simulink model "angle_led"  (R2021b)
settings: Solver=FixedStepDiscrete  StartTime=0.0  StopTime=inf  FixedStep=0.0005  RelTol=1e-3
libraries: simulink x4
settings Model: Creator=ysl  LastModifiedBy=ysl
settings OptimizationCC: DefaultParameterBehavior=Inlined  EnhancedBackFolding=on  PassReuseOutputArgsAs=Individual arguments  ZeroExternalMemoryAtStartup=off  ZeroInternalMemoryAtStartup=off  OptimizeBlockOrder=speed  DifferentSizesBufferReuse=on  OptimizationCustomize=off  EfficientTunableParamExpr=on
settings DebuggingCC: ParameterTunabilityLossMsg=error
settings SFSimCC: MATLABDynamicMemAlloc=off
settings RTWCC: Description=IFR StackLite-DualDrive Base on stm32f405RGT6  SystemTargetFile=stacklite_dualdrive.tlc  TemplateMakefile=stacklite_dualdrive.tmf  GenerateReport=on
settings CodeAppCC: ForceParamTrailComments=on  IgnoreCustomStorageClasses=off  OperatorAnnotations=on  SimulinkDataObjDesc=on  SFDataObjDesc=on  InsertBlockDesc=on
settings STFCustomTargetCC: TargetLangStandard=C99 (ISO)  MultiwordLength=256  ModelReferenceCompliant=off  CombineOutputUpdateFcns=on  ERTCustomFileBanners=on  SupportContinuousTime=off  SupportNonInlinedSFcns=off  RemoveResetFunc=on  MATLABClassNameForMDSCustomization=Simulink.SoftwareTarget.ERTCustomization  GRTInterface=off  SystemTargetFile=stacklite_dualdrive.tlc
settings ERTTargetCC: TargetLangStandard=C99 (ISO)  ModelReferenceCompliant=off  ParMdlRefBuildCompliant=off  CompOptLevelCompliant=off  ConcurrentExecutionCompliant=off  ModelStepFunctionPrototypeControlCompliant=off  CPPClassGenCompliant=off  UseToolchainInfoCompliant=off  InlinedParameterPlacement=NonHierarchical  ERTCustomFileTemplate=example_file_process.tlc

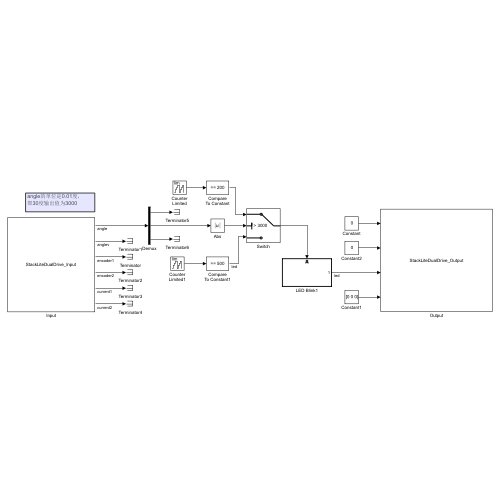
[thumbnail: Simulink's stored preview of the top-level diagram]
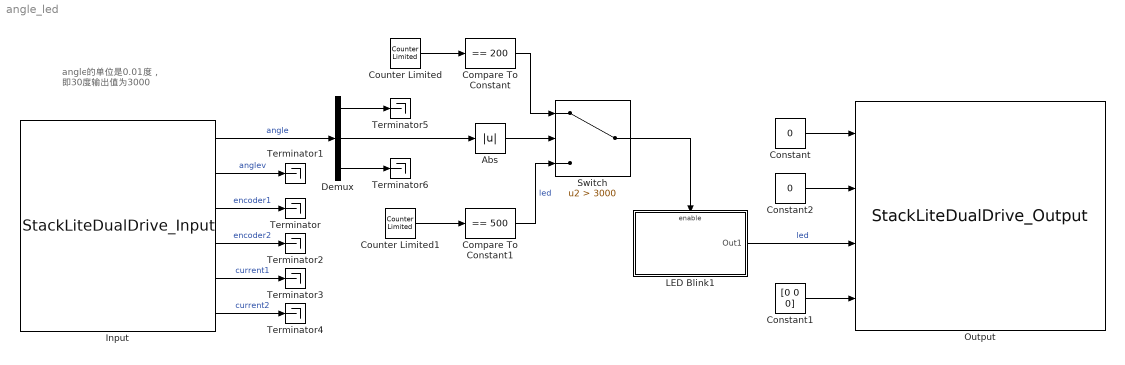
== system angle_led ==
  note: angle的单位是0.01度，
      | 即30度输出值为3000
  Abs : Abs
  Compare To Constant : simulink/Logic and Bit Operations/Compare To Constant  relop===  const=200  OutDataTypeStr=boolean
  Compare To Constant1 : simulink/Logic and Bit Operations/Compare To Constant  relop===  const=500  OutDataTypeStr=boolean
  Constant : Constant  Value=0  OutDataTypeStr=int16
  Constant1 : Constant  Value=[0 0 0]  OutDataTypeStr=uint8
  Constant2 : Constant  Value=0  OutDataTypeStr=int16
  Counter Limited : simulink/Sources/Counter Limited  uplimit=200  tsamp=-1
  Counter Limited1 : simulink/Sources/Counter Limited  uplimit=500  tsamp=-1
  Demux : Demux  Outputs=3
  Input : S-Function  Priority=0  FunctionName=StackLiteDualDrive_Input  SFunctionModules=StackLiteDualDrive_Input  SFunctionDeploymentMode=off  EnableBusSupport=off  mask(input){}
      mask help: input
      mask Help: input
  LED Blink1 : Subsystem
  Output : S-Function  Priority=255  FunctionName=StackLiteDualDrive_Output  SFunctionModules=StackLiteDualDrive_Output  SFunctionDeploymentMode=off  EnableBusSupport=off  mask(output){}
      mask help: output
      mask Help: output
  Switch : Switch  Criteria=u2 > Threshold  Threshold=3000
  Terminator{,1..6} (7 alike) : Terminator
  wires:
  Constant2/1 -> Output/2
  Compare To Constant/1 -> Switch/1
  Compare To Constant1/1 -> Switch/3  "led"
  Input/5 -> Terminator3/1  "current1"
  Input/6 -> Terminator4/1  "current2"
  Abs/1 -> Switch/2
  Demux/2 -> Abs/1
  Input/3 -> Terminator/1  "encoder1"
  Constant1/1 -> Output/4
  Input/1 -> Demux/1  "angle"
  Demux/3 -> Terminator6/1
  Constant/1 -> Output/1
  LED Blink1/1(Out1) -> Output/3  "led"
  Input/2 -> Terminator1/1  "anglev"
  Input/4 -> Terminator2/1  "encoder2"
  Switch/1 -> LED Blink1/Enable
  Counter Limited1/1 -> Compare To Constant1/1
  Counter Limited/1 -> Compare To Constant/1
  Demux/1 -> Terminator5/1

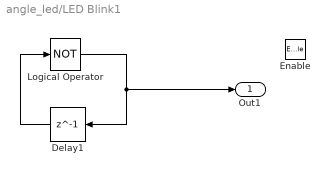
== system angle_led/LED Blink1 ==
  Enable : EnablePort
  Delay1 : Delay  DelayLength=1  InitialCondition=uint8(0)
  Logical Operator : Logic  Operator=NOT  Inputs=1  AllPortsSameDT=off  OutDataTypeStr=fixdt(0,8)
  Out1 : Outport  VectorParamsAs1DForOutWhenUnconnected=off
  wires:
  Logical Operator/1 -> Out1/1, Delay1/1
  Delay1/1 -> Logical Operator/1
